simulink model "BlochModel"  (R2016b)
settings: Solver=FixedStepAuto  StartTime=0.0  StopTime=inf  FixedStep=0.01  RelTol=1e-3
libraries: spin x1
settings Model: Creator=nzhao  LastModifiedBy=nzhao

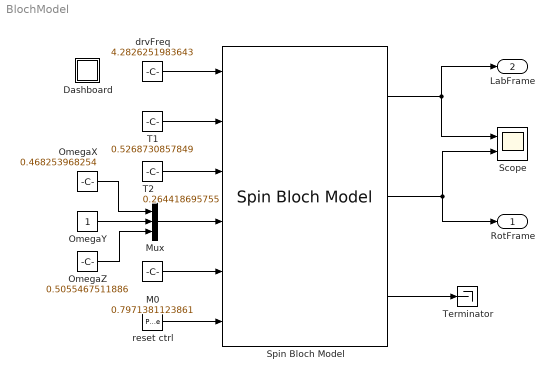
== system BlochModel ==
  Dashboard : Subsystem
  M0 : Constant  Value=0.7971381123861
  Mux : Mux  Inputs=3
  OmegaX : Constant  Value=0.468253968254
  OmegaY : Constant
  OmegaZ : Constant  Value=0.5055467511886
  Scope : Scope  NumInputPorts=2
  Spin Bloch Model : spin/Spin Bloch Model
  T1 : Constant  Value=0.5268730857849
  T2 : Constant  Value=0.264418695755
  Terminator : Terminator
  drvFreq : Constant  Value=4.2826251983643
  reset ctrl : DiscretePulseGenerator  PulseType=Time based  Period=5  PulseWidth=5
  RotFrame : Outport
  LabFrame : Outport  Port=2
  wires:
  OmegaX/1 -> Mux/1
  OmegaY/1 -> Mux/2
  OmegaZ/1 -> Mux/3
  drvFreq/1 -> Spin Bloch Model/1
  T1/1 -> Spin Bloch Model/2
  T2/1 -> Spin Bloch Model/3
  Mux/1 -> Spin Bloch Model/4
  M0/1 -> Spin Bloch Model/5
  reset ctrl/1 -> Spin Bloch Model/6
  Spin Bloch Model/1 -> LabFrame/1, Scope/1
  Spin Bloch Model/2 -> RotFrame/1, Scope/2
  Spin Bloch Model/3 -> Terminator/1

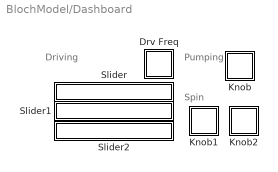
== system BlochModel/Dashboard ==
  note: Spin
  note: Pumping
  note: Driving
  Drv Freq : Subsystem  DialogController=hmiCreateDDGDialog  IsWebBlock=on  mask(MWDashboardBlock){webBlockId=11fad1a0-d078-4a93-b1f2-24675cd840d6, webBlockType=continuousknob, ShowInLibBrowser=on, ShowInitialText=on, HMISrcModelName=BlochModel}
      mask prompts: webBlockId "WebBlock Id"; webBlockType "WebBlock Type"; HMISrcModelName "Source Model"
      mask help: SimulinkHMI:dialogs:ContinuousKnobDialogDesc
      mask Help: helpview([docroot '/mapfiles/simulink.map'], 'hmi_knob')
      mask Display:
      | if strcmp(get_param(bdroot(gcb),'BlockDiagramType'), 'library')
      |     image([(matlabroot) '/toolbox/simulink/hmi/icons/ContinuousKnob.png']);
      | end
  Knob : Subsystem  DialogController=hmiCreateDDGDialog  IsWebBlock=on  mask(MWDashboardBlock){webBlockId=73ca885b-3777-40ae-9153-26abbe03700b, webBlockType=continuousknob, ShowInLibBrowser=on, ShowInitialText=on, HMISrcModelName=BlochModel}
      mask prompts: webBlockId "WebBlock Id"; webBlockType "WebBlock Type"; HMISrcModelName "Source Model"
      mask help: SimulinkHMI:dialogs:ContinuousKnobDialogDesc
      mask Help: helpview([docroot '/mapfiles/simulink.map'], 'hmi_knob')
      mask Display:
      | if strcmp(get_param(bdroot(gcb),'BlockDiagramType'), 'library')
      |     image([(matlabroot) '/toolbox/simulink/hmi/icons/ContinuousKnob.png']);
      | end
  Knob1 : Subsystem  DialogController=hmiCreateDDGDialog  IsWebBlock=on  mask(MWDashboardBlock){webBlockId=7c86e9a1-e98b-49a6-9739-53d8abf261ff, webBlockType=continuousknob, ShowInLibBrowser=on, ShowInitialText=on, HMISrcModelName=BlochModel}
      mask prompts: webBlockId "WebBlock Id"; webBlockType "WebBlock Type"; HMISrcModelName "Source Model"
      mask help: SimulinkHMI:dialogs:ContinuousKnobDialogDesc
      mask Help: helpview([docroot '/mapfiles/simulink.map'], 'hmi_knob')
      mask Display:
      | if strcmp(get_param(bdroot(gcb),'BlockDiagramType'), 'library')
      |     image([(matlabroot) '/toolbox/simulink/hmi/icons/ContinuousKnob.png']);
      | end
  Knob2 : Subsystem  DialogController=hmiCreateDDGDialog  IsWebBlock=on  mask(MWDashboardBlock){webBlockId=21515176-7d2a-4f41-995f-e1a62c466085, webBlockType=continuousknob, ShowInLibBrowser=on, ShowInitialText=on, HMISrcModelName=BlochModel}
      mask prompts: webBlockId "WebBlock Id"; webBlockType "WebBlock Type"; HMISrcModelName "Source Model"
      mask help: SimulinkHMI:dialogs:ContinuousKnobDialogDesc
      mask Help: helpview([docroot '/mapfiles/simulink.map'], 'hmi_knob')
      mask Display:
      | if strcmp(get_param(bdroot(gcb),'BlockDiagramType'), 'library')
      |     image([(matlabroot) '/toolbox/simulink/hmi/icons/ContinuousKnob.png']);
      | end
  Slider : Subsystem  DialogController=hmiCreateDDGDialog  IsWebBlock=on  mask(MWDashboardBlock){webBlockId=2b530948-c920-4ae1-9cd6-da5b9488891f, webBlockType=slider, ShowInLibBrowser=on, ShowInitialText=on, HMISrcModelName=BlochModel}
      mask prompts: webBlockId "WebBlock Id"; webBlockType "WebBlock Type"; HMISrcModelName "Source Model"
      mask help: SimulinkHMI:dialogs:SliderDialogDesc
      mask Help: helpview([docroot '/mapfiles/simulink.map'], 'hmi_slider')
      mask Display:
      | if strcmp(get_param(bdroot(gcb),'BlockDiagramType'), 'library')
      |     image([(matlabroot) '/toolbox/simulink/hmi/icons/Slider.png']);
      | end
  Slider1 : Subsystem  DialogController=hmiCreateDDGDialog  IsWebBlock=on  mask(MWDashboardBlock){webBlockId=4e9e5ef3-cf65-424b-a2c2-6c2b7a4b8921, webBlockType=slider, ShowInLibBrowser=on, ShowInitialText=on, HMISrcModelName=BlochModel}
      mask prompts: webBlockId "WebBlock Id"; webBlockType "WebBlock Type"; HMISrcModelName "Source Model"
      mask help: SimulinkHMI:dialogs:SliderDialogDesc
      mask Help: helpview([docroot '/mapfiles/simulink.map'], 'hmi_slider')
      mask Display:
      | if strcmp(get_param(bdroot(gcb),'BlockDiagramType'), 'library')
      |     image([(matlabroot) '/toolbox/simulink/hmi/icons/Slider.png']);
      | end
  Slider2 : Subsystem  DialogController=hmiCreateDDGDialog  IsWebBlock=on  mask(MWDashboardBlock){webBlockId=033e36d1-fe18-43ff-8e27-39e0f3ef90d1, webBlockType=slider, ShowInLibBrowser=on, ShowInitialText=on, HMISrcModelName=BlochModel}
      mask prompts: webBlockId "WebBlock Id"; webBlockType "WebBlock Type"; HMISrcModelName "Source Model"
      mask help: SimulinkHMI:dialogs:SliderDialogDesc
      mask Help: helpview([docroot '/mapfiles/simulink.map'], 'hmi_slider')
      mask Display:
      | if strcmp(get_param(bdroot(gcb),'BlockDiagramType'), 'library')
      |     image([(matlabroot) '/toolbox/simulink/hmi/icons/Slider.png']);
      | end

== system BlochModel/Dashboard/Drv Freq ==

== system BlochModel/Dashboard/Knob ==

== system BlochModel/Dashboard/Knob1 ==

== system BlochModel/Dashboard/Knob2 ==

== system BlochModel/Dashboard/Slider ==

== system BlochModel/Dashboard/Slider1 ==

== system BlochModel/Dashboard/Slider2 ==
